simulink model "CartPendulumLQR"  (R2019a)
settings: Solver=FixedStepAuto  StartTime=0.0  StopTime=10  RelTol=1e-3
InitFcn:
  | run Initialize.m
StopFcn:
  | run Visualization.m
undefined symbols (not defined in the file or in its folder): K, Ts, x0, xr
settings Model: Creator=visha  LastModifiedBy=visha

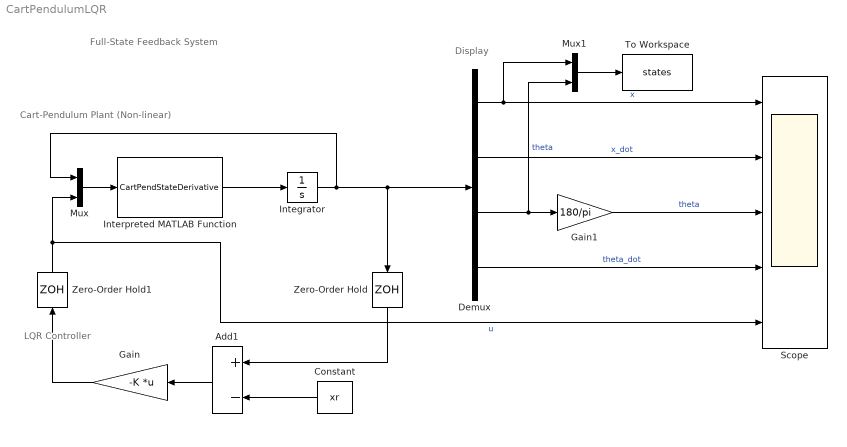
== system CartPendulumLQR ==
  note: Full-State Feedback System
  note: Display
  note: LQR Controller
  note: Cart-Pendulum Plant (Non-linear)
  Add1 : Sum  Inputs=+-
  Constant : Constant  Value=xr
  Demux : Demux
  Gain : Gain  Gain=-K  Multiplication=Matrix(K*u)
  Gain1 : Gain  Gain=180/pi
  Integrator : Integrator  InitialCondition=x0
  Interpreted MATLAB Function : MATLABFcn  MATLABFcn=CartPendStateDerivative
  Mux : Mux  Inputs=2
  Mux1 : Mux  Inputs=2
  Scope : Scope  NumInputPorts=5
  To Workspace : ToWorkspace  VariableName=states  SaveFormat=Timeseries  SampleTime=-1
  Zero-Order Hold : ZeroOrderHold  SampleTime=Ts
  Zero-Order Hold1 : ZeroOrderHold  SampleTime=Ts
  wires:
  Integrator/1 -> Mux/1, Zero-Order Hold/1, Demux/1
  Interpreted MATLAB Function/1 -> Integrator/1
  Add1/1 -> Gain/1
  Constant/1 -> Add1/2
  Mux/1 -> Interpreted MATLAB Function/1
  Demux/4 -> Scope/4  "theta_dot"
  Demux/2 -> Scope/2  "x_dot"
  Demux/1 -> Mux1/1, Scope/1  "x"
  Demux/3 -> Gain1/1, Mux1/2  "theta"
  Mux1/1 -> To Workspace/1
  Zero-Order Hold/1 -> Add1/1
  Gain/1 -> Zero-Order Hold1/1
  Zero-Order Hold1/1 -> Mux/2, Scope/5  "u"
  Gain1/1 -> Scope/3  "theta"
